simulink model "joystickcalibtest"  (Simulink 10.0)
settings: Solver=ode45  StartTime=0.0  StopTime=Inf  RelTol=1e-3  EnableMultiTasking=on
libraries: vrlib x1
settings Model: Creator=tjjlombaerts  LastModifiedBy=mauro
settings DataIOCC: LimitDataPoints=on  SignalLoggingSaveFormat=ModelDataLogs  SignalLoggingName=sigsOut
settings OptimizationCC: ExpressionDepthLimit=2147483647  InitFltsAndDblsToZero=on
settings DebuggingCC: SaveWithParameterizedLinksMsg=none  SignalResolutionControl=TryResolveAllWithWarning  MultiTaskDSMMsg=warning  MultiTaskCondExecSysMsg=none  FcnCallInpInsideContextMsg=warning  StateNameClashWarn=warning
settings HardwareCC: TargetUnknown=on

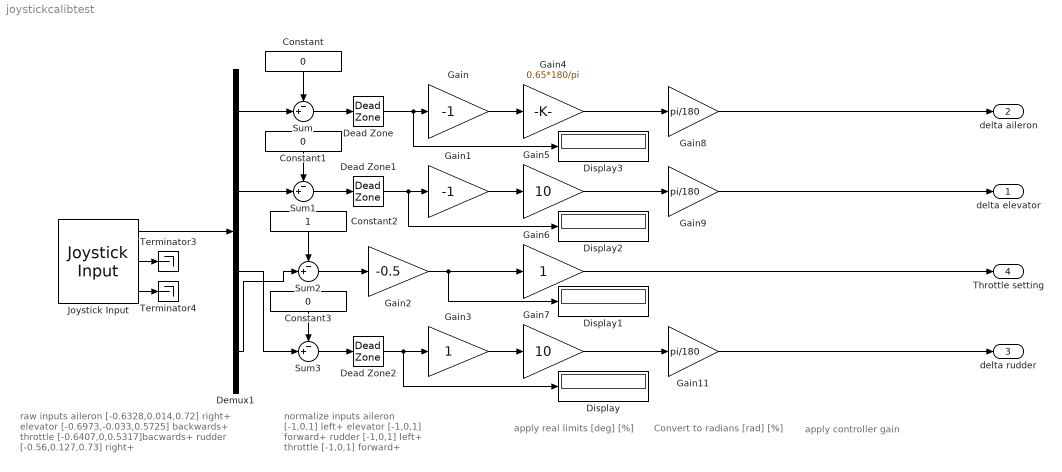
== system joystickcalibtest ==
  note: raw inputs
      | aileron [-0.6328,0.014,0.72] right+
      | elevator [-0.6973,-0.033,0.5725] backwards+
      | throttle [-0.6407,0,0.5317]bacwards+
      | rudder [-0.56,0.127,0.73] right+
  note: normalize inputs
      | aileron [-1,0,1] left+
      | elevator [-1,0,1] forward+
      | rudder [-1,0,1] left+
      | throttle [-1,0,1] forward+
  note: apply real limits
      | [deg]
      | [%]
  note: Convert to radians
      | [rad]
      | [%]
  note: apply controller
      | gain
  Constant : Constant  Value=0
  Constant1 : Constant  Value=0
  Constant2 : Constant
  Constant3 : Constant  Value=0
  Dead Zone : DeadZone  LowerValue=-0.01  UpperValue=0.01  SaturateOnIntegerOverflow=on
  Dead Zone1 : DeadZone  LowerValue=-0.02  UpperValue=0.02  SaturateOnIntegerOverflow=on
  Dead Zone2 : DeadZone  LowerValue=-0.01  UpperValue=0.01  SaturateOnIntegerOverflow=on
  Demux1 : Demux
  Display{,1..3} (4 alike) : Display
  Gain : Gain  Gain=-1  SaturateOnIntegerOverflow=on  OutDataTypeStr=Inherit: Same as input  ParamDataTypeStr=Inherit: Same as input
  Gain1 : Gain  Gain=-1  SaturateOnIntegerOverflow=on  OutDataTypeStr=Inherit: Same as input  ParamDataTypeStr=Inherit: Same as input
  Gain11 : Gain  Gain=pi/180  SaturateOnIntegerOverflow=on  OutDataTypeStr=Inherit: Same as input  ParamDataTypeStr=Inherit: Same as input
  Gain2 : Gain  Gain=-0.5  SaturateOnIntegerOverflow=on  OutDataTypeStr=Inherit: Same as input  ParamDataTypeStr=Inherit: Same as input
  Gain3 : Gain  SaturateOnIntegerOverflow=on  OutDataTypeStr=Inherit: Same as input  ParamDataTypeStr=Inherit: Same as input
  Gain4 : Gain  Gain=0.65*180/pi  SaturateOnIntegerOverflow=on  OutDataTypeStr=Inherit: Same as input  ParamDataTypeStr=Inherit: Same as input
  Gain5 : Gain  Gain=10  SaturateOnIntegerOverflow=on  OutDataTypeStr=Inherit: Same as input  ParamDataTypeStr=Inherit: Same as input
  Gain6 : Gain  SaturateOnIntegerOverflow=on  OutDataTypeStr=Inherit: Same as input  ParamDataTypeStr=Inherit: Same as input
  Gain7 : Gain  Gain=10  SaturateOnIntegerOverflow=on  OutDataTypeStr=Inherit: Same as input  ParamDataTypeStr=Inherit: Same as input
  Gain8 : Gain  Gain=pi/180  SaturateOnIntegerOverflow=on  OutDataTypeStr=Inherit: Same as input  ParamDataTypeStr=Inherit: Same as input
  Gain9 : Gain  Gain=pi/180  SaturateOnIntegerOverflow=on  OutDataTypeStr=Inherit: Same as input  ParamDataTypeStr=Inherit: Same as input
  Joystick Input : vrlib/Joystick Input  joyid=1  adjustports=on  forcefeed=off
      settings: SourceProductName=Simulink
  Sum{,1..3} (4 alike) : Sum  Inputs=-+|  SaturateOnIntegerOverflow=on
  Terminator3 : Terminator
  Terminator4 : Terminator
  delta elevator : Outport
  delta aileron : Outport  Port=2
  delta rudder : Outport  Port=3
  Throttle setting : Outport  Port=4
  wires:
  Joystick Input/1 -> Demux1/1
  Joystick Input/2 -> Terminator3/1
  Joystick Input/3 -> Terminator4/1
  Demux1/1 -> Sum/2
  Constant/1 -> Sum/1
  Constant1/1 -> Sum1/1
  Demux1/2 -> Sum1/2
  Constant2/1 -> Sum2/1
  Constant3/1 -> Sum3/1
  Sum/1 -> Dead Zone/1
  Gain/1 -> Gain4/1
  Sum1/1 -> Dead Zone1/1
  Gain1/1 -> Gain5/1
  Sum2/1 -> Gain2/1
  Sum3/1 -> Dead Zone2/1
  Gain3/1 -> Gain7/1
  Gain4/1 -> Gain8/1
  Gain5/1 -> Gain9/1
  Gain6/1 -> Throttle setting/1
  Gain7/1 -> Gain11/1
  Gain8/1 -> delta aileron/1
  Gain9/1 -> delta elevator/1
  Gain11/1 -> delta rudder/1
  Gain2/1 -> Gain6/1, Display1/1
  Demux1/3 -> Sum3/2
  Demux1/4 -> Sum2/2
  Dead Zone/1 -> Gain/1, Display3/1
  Dead Zone1/1 -> Gain1/1, Display2/1
  Dead Zone2/1 -> Gain3/1, Display/1
